simulink model "Controller_empty"  (R2019b)
settings: Solver=VariableStepAuto  StartTime=0.0  StopTime=10.0  RelTol=1e-3
undefined symbols (not defined in the file or in its folder): UseUserDefinedBallReference, UseUserDefinedPlateReference
settings Model: Creator=Duin home  LastModifiedBy=Duin home

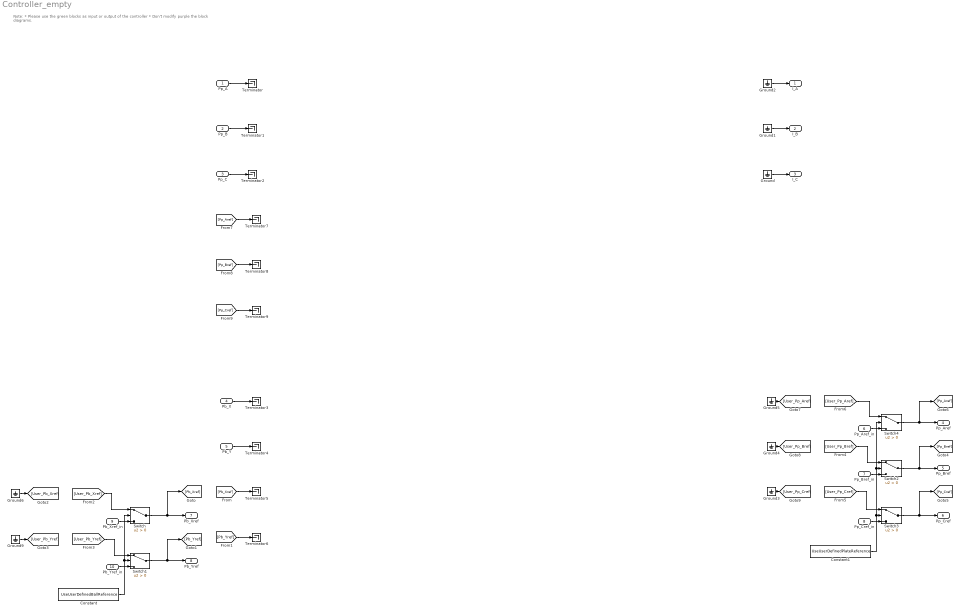
== system Controller_empty ==
  note: Note:
      | * Please use the green blocks as input or output of the controller
      | * Don't modify purple the block diagrams.
  Pp_A : Inport
  Pp_B : Inport  Port=2
  Pp_C : Inport  Port=3
  Pb_X : Inport  Port=4
  Pb_Y : Inport  Port=5
  Pp_Aref_in : Inport  Port=6
  Pp_Bref_in : Inport  Port=7
  Pp_Cref_in : Inport  Port=8
  Pb_Xref_in : Inport  Port=9
  Pb_Yref_in : Inport  Port=10
  Constant : Constant  Value=UseUserDefinedBallReference
  Constant1 : Constant  Value=UseUserDefinedPlateReference
  Ground{,1..6,9} (8 alike) : Ground
  Switch{,1..4} (5 alike) : Switch  Criteria=u2 > Threshold
  Terminator{,1..9} (10 alike) : Terminator
  I_A : Outport
  I_B : Outport  Port=2
  I_C : Outport  Port=3
  Pp_Aref : Outport  Port=4
  Pp_Bref : Outport  Port=5
  Pp_Cref : Outport  Port=6
  Pb_Xref : Outport  Port=7
  Pb_Yref : Outport  Port=8
  wires:
  Pp_A/1 -> Terminator/1
  Pp_B/1 -> Terminator1/1
  Pp_C/1 -> Terminator2/1
  Pb_X/1 -> Terminator3/1
  Pb_Y/1 -> Terminator4/1
  Ground/1 -> I_C/1
  Ground1/1 -> I_B/1
  Ground2/1 -> I_A/1
  Ground3/1 -> [User_Pp_Cref]
  Ground4/1 -> [User_Pp_Bref]
  Ground5/1 -> [User_Pp_Aref]
  Pb_Xref_in/1 -> Switch/3
  Pb_Yref_in/1 -> Switch1/3
  Switch1/1 -> [Pb_Yref], Pb_Yref/1
  Switch/1 -> [Pb_Xref], Pb_Xref/1
  [User_Pb_Xref] -> Switch/1
  [User_Pb_Yref] -> Switch1/1
  Constant/1 -> Switch/2, Switch1/2
  Ground9/1 -> [User_Pb_Yref]
  [Pb_Yref] -> Terminator6/1
  [Pb_Xref] -> Terminator5/1
  Pp_Bref_in/1 -> Switch2/3
  [User_Pp_Bref] -> Switch2/1
  Switch3/1 -> [Pp_Cref], Pp_Cref/1
  Switch2/1 -> [Pp_Bref], Pp_Bref/1
  Pp_Cref_in/1 -> Switch3/3
  Constant1/1 -> Switch4/2, Switch2/2, Switch3/2
  [User_Pp_Cref] -> Switch3/1
  [User_Pp_Aref] -> Switch4/1
  Pp_Aref_in/1 -> Switch4/3
  Switch4/1 -> [Pp_Aref], Pp_Aref/1
  [Pp_Bref] -> Terminator8/1
  [Pp_Aref] -> Terminator7/1
  [Pp_Cref] -> Terminator9/1
  Ground6/1 -> [User_Pb_Xref]
